simulink model "VCU_SW"  (R2020b)
settings: Solver=FixedStepDiscrete  StartTime=0.0  StopTime=inf  FixedStep=1e-2  RelTol=1e-3
PreLoadFcn:
  | RTWConfigurationCB('preloadfcn', bdroot);
InitFcn:
  | loadvar_ttc500
undefined symbols (not defined in the file or in its folder): BrkPedalTypes, CabMovModeTypes, cFuseTempSensAcc_X, cFuseTempSensAcc_Y, cFuseTempSensVal_X, cFuseTempSensVal_Y, cTMSTempSensVal_X, cTMSTempSensVal_Y, cTransferCaseSpeedRatio, diag_state, DoorsPositionTypes, dP_filter_Y, DriverOccClassSystemTypes, ErrorValueTypes, fatal_error_callback, IO_ADC_NO_RANGE, LadderStatusTypes, pAnalogCabRotSensAcc, pAnalogCabRotSensMaxVolt, pAnalogCabRotSensMinVolt, pAnalogCabRotSensRange, pAnalogCabRotSensZeroVolt, pBrkActivePress, pCabTiltSensAcc, pCabTiltSensMaxCur, pCabTiltSensMinCur, pDistanceCorrection, pECANManual_BPNEnable, pECANManual_BPNEnabler_Flag, pFilterSensAccRes, pHDirMaxDiffFrq, pHDirSensHighLvl, pHDirSensLowLvl, pMainGearRatio, pMaxFilterSensRes, pMaxFirstPedalSensValue, pMaxFuseTempSensRes, pMaxPressLoss, pMaxPressSensCurrent, pMaxPressValue, pMaxPressValueHydMotAndPump, pMaxPressValueParkDrain, pMaxSecondPedalSensValue, pMaxTempSensVoltage, pMaxTempValue, pMaxTMSTempSensRes, pMinFilterSensRes, pMinFirstPedalSensValue, pMinFuseTempSensRes, pMinPressLoss, pMinPressSensCurrent, pMinPressValue, pMinSecondPedalSensValue, pMinTempSensVoltage, pMinTempValue, pMinTMSTempSensRes, pMotorRingTeethNum, pPedalSensAccuracyPct, pPedalSensAccuracyVolt, pPressLossTreshhold ... (+20)
libraries: TTlibrary x271, canmsglib x128, simulink x88
(part 8 of 17)

== system VCU_SW/OutputLayer/OutputNetwork/OutputCCAN/SetCCAN100msec ==
  function : TriggerPort  TriggerType=function-call  VariantControl=Variant
  CANPack_DCDC_IN_Control : canmsglib/CAN Pack  Commented=on  CANdbFile=C:\Users\shevchenko\Desktop\HerculesLittle\HerculesLittle\database\ElectricCAN.dbc  MsgList=(none)  MsgName=DCDC_IN_Control  MsgIDType=Extended (29-bit identifier)  MsgIdentifier=73  MsgLength=8  Remote=off  ApplyMinMax=off  BusOutput=on  SignalInfo={'BPN_Enable','0','1','LE','unsigned','Standard','0','1','0','0','1'}
      settings: SourceProductBaseCode=ME,XP,VN  DataFormat=CANdb specified signals
  CANPack_DCDC_IN_Control1 : canmsglib/CAN Pack  Commented=on  MsgList=(none)  MsgName=ETC2  MsgIDType=Extended (29-bit identifier)  MsgIdentifier=418383354  MsgLength=8  Remote=off  ApplyMinMax=off  BusOutput=on  SignalInfo={ 'Transmission_Actual_Gear_Ratio', '8', '16', 'LE', 'unsigned', 'Standard', '0', '0.001', '0', '0', '64.255'; 'Transmission_Current_Gear', '24', '8', 'LE', 'unsigned', 'Standard', '0', '1', '-125', '-125', '125'; 'Transmission_Current_Range', '48', '16', 'LE', 'unsigned', 'Standard', '0', '1', '0', '0', '65535'; 'Transmission_Requested_Range', '32', '16', 'LE', 'unsigned', 'Standard', '0', '1', '0', '0', '65535'; 'Transmission_Selected_Gear', '0', '8', 'LE', 'unsigned', 'Standard', '0', '1', '-125', '-125', '125' }
      settings: SourceProductBaseCode=ME,XP,VN  DataFormat=manually specified signals
  CCVS1 : Subsystem
  Cabine Angles : Subsystem
  "Cabine Status " : Subsystem
  Constant31 : Constant  Commented=on  Value=pECANManual_BPNEnabler_Flag
  Constant32 : Constant  Commented=on  Value=pECANManual_BPNEnable
  Data Store Read : DataStoreRead  Commented=on  DataStoreName=OutputNetworkData  DataStoreElements=DevicesControllerData.ovc_permission
  Data Store Read1 : DataStoreRead  Commented=on  DataStoreName=OutputNetworkData  DataStoreElements=DevicesControllerData.ovc_permission
  EBC1 : Subsystem
  ETC2 : Subsystem
  ETC7 : Subsystem
  "Fuel Filter Heater Status " : Subsystem
  FuelUsingOEM : Subsystem
  MATLAB Function6 : MATLAB Function  Commented=on  TreatAsAtomicUnit=on
  Multiport Switch5 : MultiPortSwitch  Commented=on  DataPortOrder=Zero-based contiguous  Inputs=2  zeroidx=on
  Terminator : Terminator  Commented=on
  Terminator1 : Terminator  Commented=on
  VD : Subsystem
  "VLVCMD_ MANIP_TABLE " : Subsystem
  transmit_message_dcdc_in_control : TTlibrary/CAN/transmit_message_name  Commented=on  channel=IO_CAN_CHANNEL_0  id_format=IO_CAN_STD_FRAME  retranslation=off  io_error=on  sample_time=-1
      settings: SourceProductName=TT control 500 series
  transmit_message_dcdc_in_control1 : TTlibrary/CAN/transmit_message_name  Commented=on  channel=IO_CAN_CHANNEL_1  id_format=IO_CAN_STD_FRAME  retranslation=off  io_error=on  sample_time=-1
      settings: SourceProductName=TT control 500 series
  wires:
  Data Store Read1/1 -> CANPack_DCDC_IN_Control1/1
  transmit_message_dcdc_in_control1/1 -> Terminator1/1  "error_tx_transmit_message_dcdc_in_control1"
  CANPack_DCDC_IN_Control1/1 -> transmit_message_dcdc_in_control1/1
  Data Store Read/1 -> MATLAB Function6/1(input)
  transmit_message_dcdc_in_control/1 -> Terminator/1  "error_tx_transmit_message_dcdc_in_control"
  MATLAB Function6/1(value) -> Multiport Switch5/2
  Multiport Switch5/1 -> CANPack_DCDC_IN_Control/1
  Constant32/1 -> Multiport Switch5/3
  CANPack_DCDC_IN_Control/1 -> transmit_message_dcdc_in_control/1
  Constant31/1 -> Multiport Switch5/1

== system VCU_SW/OutputLayer/OutputNetwork/OutputCCAN/SetCCAN10msec ==
  function : TriggerPort  TriggerType=function-call  VariantControl=Variant

== system VCU_SW/OutputLayer/OutputNetwork/OutputCCAN/SetCCAN500msec ==
  function : TriggerPort  TriggerType=function-call  VariantControl=Variant
  Brake_circuits_manip_press : Subsystem
  CANPack_DCDC_IN_Control : canmsglib/CAN Pack  Commented=on  CANdbFile=C:\Users\shevchenko\Desktop\HerculesLittle\HerculesLittle\database\ElectricCAN.dbc  MsgList=(none)  MsgName=DCDC_IN_Control  MsgIDType=Extended (29-bit identifier)  MsgIdentifier=73  MsgLength=8  Remote=off  ApplyMinMax=off  BusOutput=on  SignalInfo={'BPN_Enable','0','1','LE','unsigned','Standard','0','1','0','0','1'}
      settings: SourceProductBaseCode=ME,XP,VN  DataFormat=CANdb specified signals
  CANPack_DCDC_IN_Control1 : canmsglib/CAN Pack  Commented=on  MsgList=(none)  MsgName=ETC2  MsgIDType=Extended (29-bit identifier)  MsgIdentifier=418383354  MsgLength=8  Remote=off  ApplyMinMax=off  BusOutput=on  SignalInfo={ 'Transmission_Actual_Gear_Ratio', '8', '16', 'LE', 'unsigned', 'Standard', '0', '0.001', '0', '0', '64.255'; 'Transmission_Current_Gear', '24', '8', 'LE', 'unsigned', 'Standard', '0', '1', '-125', '-125', '125'; 'Transmission_Current_Range', '48', '16', 'LE', 'unsigned', 'Standard', '0', '1', '0', '0', '65535'; 'Transmission_Requested_Range', '32', '16', 'LE', 'unsigned', 'Standard', '0', '1', '0', '0', '65535'; 'Transmission_Selected_Gear', '0', '8', 'LE', 'unsigned', 'Standard', '0', '1', '-125', '-125', '125' }
      settings: SourceProductBaseCode=ME,XP,VN  DataFormat=manually specified signals
  Constant31 : Constant  Commented=on  Value=pECANManual_BPNEnabler_Flag
  Constant32 : Constant  Commented=on  Value=pECANManual_BPNEnable
  Data Store Read : DataStoreRead  Commented=on  DataStoreName=OutputNetworkData  DataStoreElements=DevicesControllerData.ovc_permission
  Data Store Read1 : DataStoreRead  Commented=on  DataStoreName=OutputNetworkData  DataStoreElements=DevicesControllerData.ovc_permission
  EAC1 : Subsystem
  "EFL/P1 " : Subsystem
  EFL/P12 : Subsystem  Commented=on
  MATLAB Function6 : MATLAB Function  Commented=on  TreatAsAtomicUnit=on
  Multiport Switch5 : MultiPortSwitch  Commented=on  DataPortOrder=Zero-based contiguous  Inputs=2  zeroidx=on
  Terminator : Terminator  Commented=on
  Terminator1 : Terminator  Commented=on
  transmit_message_dcdc_in_control : TTlibrary/CAN/transmit_message_name  Commented=on  channel=IO_CAN_CHANNEL_0  id_format=IO_CAN_STD_FRAME  retranslation=off  io_error=on  sample_time=-1
      settings: SourceProductName=TT control 500 series
  transmit_message_dcdc_in_control1 : TTlibrary/CAN/transmit_message_name  Commented=on  channel=IO_CAN_CHANNEL_1  id_format=IO_CAN_STD_FRAME  retranslation=off  io_error=on  sample_time=-1
      settings: SourceProductName=TT control 500 series
  wires:
  transmit_message_dcdc_in_control1/1 -> Terminator1/1  "error_tx_transmit_message_dcdc_in_control1"
  Data Store Read1/1 -> CANPack_DCDC_IN_Control1/1
  CANPack_DCDC_IN_Control1/1 -> transmit_message_dcdc_in_control1/1
  Data Store Read/1 -> MATLAB Function6/1(input)
  transmit_message_dcdc_in_control/1 -> Terminator/1  "error_tx_transmit_message_dcdc_in_control"
  MATLAB Function6/1(value) -> Multiport Switch5/2
  Multiport Switch5/1 -> CANPack_DCDC_IN_Control/1
  Constant32/1 -> Multiport Switch5/3
  CANPack_DCDC_IN_Control/1 -> transmit_message_dcdc_in_control/1
  Constant31/1 -> Multiport Switch5/1

== system VCU_SW/OutputLayer/OutputNetwork/OutputCCAN/SetCCAN50msec ==
  function : TriggerPort  TriggerType=function-call  VariantControl=Variant
  EEC1 : Subsystem
  EEC2 : Subsystem

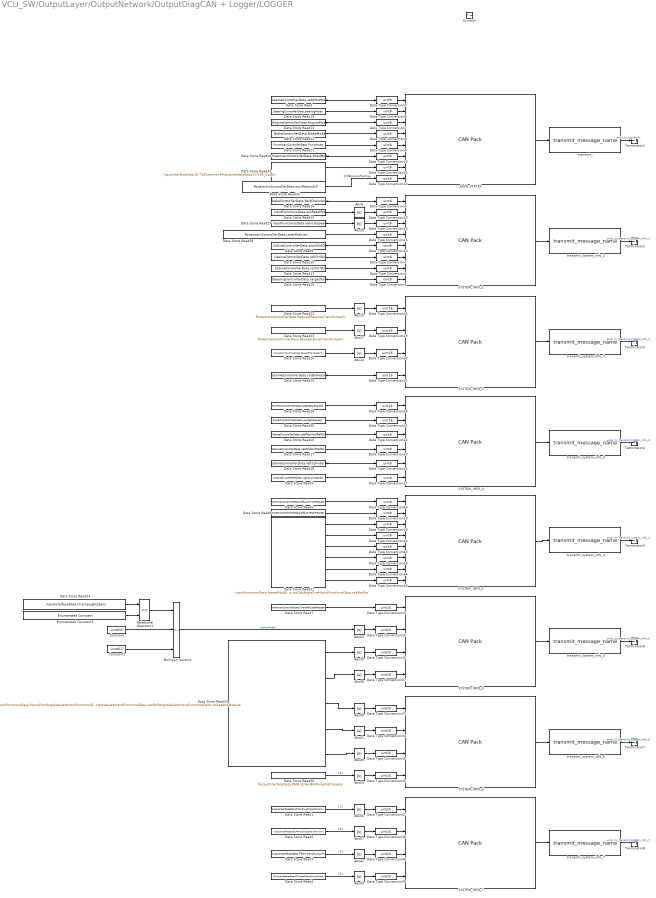
== system VCU_SW/OutputLayer/OutputNetwork/OutputDiagCAN + Logger/LOGGER ==
  function : TriggerPort  TriggerType=function-call  VariantControl=Variant
  ALGO_STATES : canmsglib/CAN Pack  MsgList=(none)  MsgName=ALGO_STATES  MsgIDType=Extended (29-bit identifier)  MsgIdentifier=419385594  MsgLength=8  Remote=off  ApplyMinMax=off  BusOutput=on  SignalInfo={ 'ALGO_MODE_1', '56', '8', 'LE', 'unsigned', 'Standard', '0', '1', '0', '0', '255'; 'ALGO_MODE_2', '48', '8', 'LE', 'unsigned', 'Standard', '0', '1', '0', '0', '255'; 'ALGO_MODE_3', '40', '8', 'LE', 'unsigned', 'Standard', '0', '1', '0', '0', '255'; 'ALGO_MODE_4', '32', '8', 'LE', 'unsigned', 'Standard', '0', '1', '0', '0', '255'; 'ALGO_MODE_5', '24', '8', 'LE', 'unsigned', 'Standard', '0', '1', '0', '0', '255'; 'ALGO_MODE_6', '16', '8', 'LE', 'unsigned', 'Standard', '0', '1', '0', '0', '255'; 'ALGO_MODE_7', '8', '8', 'LE', 'unsigned', 'Standard', '0', '1', '0', '0', '255'; 'ALGO_MODE_8', '0', '8', 'LE', 'unsigned', 'Standard', '0', '1', '0', '0', '255' }
      settings: SourceProductBaseCode=ME,XP,VN  DataFormat=manually specified signals
  Abs{9..10,16..17,24,34..35,40..43,49..50,56..57,63} (16 alike) : Abs
  Constant : Constant  Value=uint8(0)
  Constant1 : Constant  Value=uint8(1)
  Data Store Read : DataStoreRead  DataStoreName=CabineControllerData  DataStoreElements=CabineControllerData.cabMovMode
  Data Store Read1 : DataStoreRead  DataStoreName=OutputInterfaceData  DataStoreElements=OutputInterfaceData.PWM.driveTransPumpVlv
  Data Store Read10 : DataStoreRead  DataStoreName=CabineControllerData  DataStoreElements=CabineControllerData.rollCtrlDir
  Data Store Read11 : DataStoreRead  DataStoreName=CabineControllerData  DataStoreElements=CabineControllerData.rotCtrlDir
  Data Store Read12 : DataStoreRead  DataStoreName=EngineControllerData  DataStoreElements=EngineControllerData.EngineMode
  Data Store Read13 : DataStoreRead  DataStoreName=BrakeControllerData  DataStoreElements=BrakeControllerData.BrakeMode
  Data Store Read14 : DataStoreRead  DataStoreName=BrakeControllerData  DataStoreElements=BrakeControllerData.ParkDrainValve
  Data Store Read15 : DataStoreRead  DataStoreName=InputFunctionsData  DataStoreElements=InputFunctionsData.accPedalPos
  Data Store Read16 : DataStoreRead  DataStoreName=CabineControllerData  DataStoreElements=CabineControllerData.cabPitchHullRefDir
  Data Store Read17 : DataStoreRead  DataStoreName=CabineControllerData  DataStoreElements=CabineControllerData.cabRollHullRefDir
  Data Store Read18 : DataStoreRead  DataStoreName=CabineControllerData  DataStoreElements=CabineControllerData.leftCylinderDir
  Data Store Read19 : DataStoreRead  DataStoreName=SteeringControllerData  DataStoreElements=SteeringControllerData.steeringMode
  Data Store Read2 : DataStoreRead  DataStoreName=OutputInterfaceData  DataStoreElements=OutputInterfaceData.PWM.reverseTransPumpVlv
  Data Store Read20 : DataStoreRead  DataStoreName=PowertrainControllerData  DataStoreElements=PowertrainControllerData.RoadMode
  Data Store Read21 : DataStoreRead  DataStoreName=PowertrainControllerData  DataStoreElements=PowertrainControllerData.PumpMode
  Data Store Read22 : DataStoreRead  DataStoreName=PowertrainControllerData  DataStoreElements=PowertrainControllerData.RequestReverseTransPumpVlv
  Data Store Read23 : DataStoreRead  DataStoreName=PowertrainControllerData  DataStoreElements=PowertrainControllerData.RequestDriveTransPumpVlv
  Data Store Read24 : DataStoreRead  DataStoreName=PowertrainControllerData  DataStoreElements=PowertrainControllerData.RequestTransMotorVlv
  Data Store Read25 : DataStoreRead  DataStoreName=CabineControllerData  DataStoreElements=CabineControllerData.rotBrakeCmd
  Data Store Read26 : DataStoreRead  DataStoreName=SteeringControllerData  DataStoreElements=SteeringControllerData.targetValve
  Data Store Read27 : DataStoreRead  DataStoreName=InputFunctionsData  DataStoreElements=InputFunctionsData.vehicleSpeed
  Data Store Read28 : DataStoreRead  DataStoreName=PowertrainControllerData  DataStoreElements=PowertrainControllerData.LeverPosition
  Data Store Read29 : DataStoreRead  DataStoreName=PowertrainControllerData  DataStoreElements=PowertrainControllerData.UpperGearRequest
  Data Store Read3 : DataStoreRead  DataStoreName=OutputInterfaceData  DataStoreElements=OutputInterfaceData.PWM.transPumpVlv
  Data Store Read30 : DataStoreRead  DataStoreName=PowertrainControllerData  DataStoreElements=PowertrainControllerData.LowGearRequest
  Data Store Read31 : DataStoreRead  DataStoreName=InputFunctionsData  DataStoreElements=InputFunctionsData.framePitchAngleDir#InputFunctionsData.frameRollAngleDir#InputFunctionsData.cabPitchAngleDir#InputFunctionsData.cabRollAngleDir#InputFunctionsData.rotCabAngleDir#InputFunctionsData.cabRotPos
  Data Store Read32 : DataStoreRead  DataStoreName=InputFunctionsData  DataStoreElements=InputFunctionsData.framePitchAngleValue#InputFunctionsData.frameRollAngleValue#InputFunctionsData.cabPitchAngleValue#InputFunctionsData.cabRollAngleValue#InputFunctionsData.rotCabAngleValue
  Data Store Read33 : DataStoreRead  DataStoreName=InputInterfaceData  DataStoreElements=InputInterfaceData.DI.T15Common#InputInterfaceData.DI.T50_Supply
  Data Store Read34 : DataStoreRead  DataStoreName=InputInterfaceData  DataStoreElements=InputInterfaceData.DI.stopLightsSens
  Data Store Read35 : DataStoreRead  DataStoreName=PowertrainControllerData  DataStoreElements=PowertrainControllerData.movRestrictLP
  Data Store Read36 : DataStoreRead  DataStoreName=OutputInterfaceData  DataStoreElements=OutputInterfaceData.PWM.strAndBrkPumpDistrSupply
  Data Store Read4 : DataStoreRead  DataStoreName=OutputInterfaceData  DataStoreElements=OutputInterfaceData.PWM.techEquipPumpSupply
  Data Store Read5 : DataStoreRead  DataStoreName=PowertrainControllerData  DataStoreElements=PowertrainControllerData.DiffLockFrontRequest
  Data Store Read6 : DataStoreRead  DataStoreName=PowertrainControllerData  DataStoreElements=PowertrainControllerData.DiffLockRearRequest
  Data Store Read7 : DataStoreRead  DataStoreName=PowertrainControllerData  DataStoreElements=PowertrainControllerData.TransferCaseRequest
  Data Store Read8 : DataStoreRead  DataStoreName=CabineControllerData  DataStoreElements=CabineControllerData.pitchCtrlDir
  Data Store Read9 : DataStoreRead  DataStoreName=CabineControllerData  DataStoreElements=CabineControllerData.rightCylinderDir
  Data Type Conversion{1..20,22..24,42..46} (28 alike) : DataTypeConversion  OutDataTypeStr=uint8
  Data Type Conversion{21,25..41} (18 alike) : DataTypeConversion  OutDataTypeStr=uint16
  Enumerated Constant5 : simulink/Sources/Enumerated Constant  OutDataTypeStr=Enum: StateModeTypes  Value=StateModeTypes.STT_ENABLE  SampleTime=inf
  Multiport Switch2 : MultiPortSwitch  DataPortOrder=Zero-based contiguous  Inputs=2  zeroidx=on
  Relational Operator1 : RelationalOperator  Operator===  OutDataTypeStr=boolean  RndMeth=Simplest
  SYSTEM_INFO_1 : canmsglib/CAN Pack  MsgList=(none)  MsgName=SYSTEM_INFO_1  MsgIDType=Extended (29-bit identifier)  MsgIdentifier=419387642  MsgLength=8  Remote=off  ApplyMinMax=off  BusOutput=on  SignalInfo={ 'system_info_1_1', '0', '8', 'LE', 'unsigned', 'Standard', '0', '1', '0', '0', '255'; 'system_info_1_2', '8', '8', 'LE', 'unsigned', 'Standard', '0', '1', '0', '0', '255'; 'system_info_1_3', '16', '8', 'LE', 'unsigned', 'Standard', '0', '1', '0', '0', '255'; 'system_info_1_4', '24', '8', 'LE', 'unsigned', 'Standard', '0', '1', '0', '0', '255'; 'system_info_1_5', '32', '8', 'LE', 'unsigned', 'Standard', '0', '1', '0', '0', '255'; 'system_info_1_6', '40', '8', 'LE', 'unsigned', 'Standard', '0', '1', '0', '0', '255'; 'system_info_1_7', '48', '8', 'LE', 'unsigned', 'Standard', '0', '1', '0', '0', '255'; 'system_info_1_8', '56', '8', 'LE', 'unsigned', 'Standard', '0', '1', '0', '0', '255' }
      settings: SourceProductBaseCode=ME,XP,VN  DataFormat=manually specified signals
  SYSTEM_INFO_2 : canmsglib/CAN Pack  MsgList=(none)  MsgName=SYSTEM_INFO_2  MsgIDType=Extended (29-bit identifier)  MsgIdentifier=419387898  MsgLength=8  Remote=off  ApplyMinMax=off  BusOutput=on  SignalInfo={ 'system_info_2_1', '0', '16', 'LE', 'unsigned', 'Standard', '0', '1', '0', '0', '65535'; 'system_info_2_2', '16', '16', 'LE', 'unsigned', 'Standard', '0', '1', '0', '0', '65535'; 'system_info_2_3', '32', '16', 'LE', 'unsigned', 'Standard', '0', '1', '0', '0', '65535'; 'system_info_2_4', '48', '16', 'LE', 'unsigned', 'Standard', '0', '1', '0', '0', '65535' }
      settings: SourceProductBaseCode=ME,XP,VN  DataFormat=manually specified signals
  SYSTEM_INFO_3 : canmsglib/CAN Pack  MsgList=(none)  MsgName=SYSTEM_INFO_3  MsgIDType=Extended (29-bit identifier)  MsgIdentifier=419389690  MsgLength=8  Remote=off  ApplyMinMax=off  BusOutput=on  SignalInfo={ 'system_info_3_1', '0', '16', 'LE', 'unsigned', 'Standard', '0', '1', '0', '0', '65535'; 'system_info_3_3', '16', '16', 'LE', 'unsigned', 'Standard', '0', '1', '0', '0', '65535'; 'system_info_3_5', '32', '8', 'LE', 'unsigned', 'Standard', '0', '1', '0', '0', '255'; 'system_info_3_6', '40', '8', 'LE', 'unsigned', 'Standard', '0', '1', '0', '0', '255'; 'system_info_3_7', '48', '8', 'LE', 'unsigned', 'Standard', '0', '1', '0', '0', '255'; 'system_info_3_8', '56', '8', 'LE', 'unsigned', 'Standard', '0', '1', '0', '0', '255' }
      settings: SourceProductBaseCode=ME,XP,VN  DataFormat=manually specified signals
  SYSTEM_INFO_4 : canmsglib/CAN Pack  MsgList=(none)  MsgName=SYSTEM_INFO_4  MsgIDType=Extended (29-bit identifier)  MsgIdentifier=419389946  MsgLength=8  Remote=off  ApplyMinMax=off  BusOutput=on  SignalInfo={ 'system_info_4_1', '0', '8', 'LE', 'unsigned', 'Standard', '0', '1', '0', '0', '255'; 'system_info_4_2', '8', '8', 'LE', 'unsigned', 'Standard', '0', '1', '0', '0', '255'; 'system_info_4_3', '16', '8', 'LE', 'unsigned', 'Standard', '0', '1', '0', '0', '255'; 'system_info_4_4', '24', '8', 'LE', 'unsigned', 'Standard', '0', '1', '0', '0', '255'; 'system_info_4_5', '32', '8', 'LE', 'unsigned', 'Standard', '0', '1', '0', '-Inf', 'Inf'; 'system_info_4_6', '40', '8', 'LE', 'unsigned', 'Standard', '0', '1', '0', '-Inf', 'Inf'; 'system_info_4_7', '48', '8', 'LE', 'unsigned', 'Standard', '0', '1', '0', '-Inf', 'Inf'; 'system_info_4_8', '56', '8', 'LE', 'unsigned', 'Standard', '0', '1', '0', '-Inf', 'Inf' }
      settings: SourceProductBaseCode=ME,XP,VN  DataFormat=manually specified signals
  SYSTEM_INFO_5 : canmsglib/CAN Pack  MsgList=(none)  MsgName=SYSTEM_INFO_5  MsgIDType=Extended (29-bit identifier)  MsgIdentifier=419390202  MsgLength=8  Remote=off  ApplyMinMax=off  BusOutput=on  SignalInfo={ 'system_info_5_1', '0', '16', 'LE', 'unsigned', 'Standard', '0', '1', '0', '0', '65535'; 'system_info_5_2', '16', '16', 'LE', 'unsigned', 'Standard', '0', '1', '0', '0', '65535'; 'system_info_5_3', '32', '16', 'LE', 'unsigned', 'Standard', '0', '1', '0', '0', '65535'; 'system_info_5_4', '48', '16', 'LE', 'unsigned', 'Standard', '0', '1', '0', '0', '65535' }
      settings: SourceProductBaseCode=ME,XP,VN  DataFormat=manually specified signals
  SYSTEM_INFO_6 : canmsglib/CAN Pack  MsgList=(none)  MsgName=SYSTEM_INFO_6  MsgIDType=Extended (29-bit identifier)  MsgIdentifier=419390458  MsgLength=8  Remote=off  ApplyMinMax=off  BusOutput=on  SignalInfo={ 'system_info_6_1', '0', '16', 'LE', 'unsigned', 'Standard', '0', '1', '0', '0', '65535'; 'system_info_6_2', '16', '16', 'LE', 'unsigned', 'Standard', '0', '1', '0', '0', '65535'; 'system_info_6_3', '32', '16', 'LE', 'unsigned', 'Standard', '0', '1', '0', '0', '65535'; 'system_info_6_4', '48', '16', 'LE', 'unsigned', 'Standard', '0', '1', '0', '0', '65535' }
      settings: SourceProductBaseCode=ME,XP,VN  DataFormat=manually specified signals
  SYSTEM_INFO_7 : canmsglib/CAN Pack  MsgList=(none)  MsgName=SYSTEM_INFO_7  MsgIDType=Extended (29-bit identifier)  MsgIdentifier=419391226  MsgLength=8  Remote=off  ApplyMinMax=off  BusOutput=on  SignalInfo={ 'system_info_7_1', '0', '16', 'LE', 'unsigned', 'Standard', '0', '1', '0', '0', '65535'; 'system_info_7_2', '16', '16', 'LE', 'unsigned', 'Standard', '0', '1', '0', '0', '65535'; 'system_info_7_3', '32', '16', 'LE', 'unsigned', 'Standard', '0', '1', '0', '0', '65535'; 'system_info_7_4', '48', '16', 'LE', 'unsigned', 'Standard', '0', '1', '0', '0', '65535' }
      settings: SourceProductBaseCode=ME,XP,VN  DataFormat=manually specified signals
  Terminator{1..8} (8 alike) : Terminator
  transmit_ : TTlibrary/CAN/transmit_message_name  channel=IO_CAN_CHANNEL_6  id_format=IO_CAN_EXT_FRAME  retranslation=off  io_error=on  sample_time=-1
      settings: SourceProductName=TT control 500 series
  transmit_system_info_{1..7} (7 alike) : TTlibrary/CAN/transmit_message_name  channel=IO_CAN_CHANNEL_6  id_format=IO_CAN_EXT_FRAME  retranslation=off  io_error=on  sample_time=-1
      settings: SourceProductName=TT control 500 series
  wires:
  Data Type Conversion6/1 -> ALGO_STATES/2
  Data Store Read13/1 -> Data Type Conversion8/1
  Data Store Read12/1 -> Data Type Conversion7/1
  Data Store Read33/1 -> Data Type Conversion11/1
  Data Store Read19/1 -> Data Type Conversion6/1
  Data Store Read/1 -> Data Type Conversion3/1
  Data Store Read20/1 -> Data Type Conversion10/1
  Data Store Read21/1 -> Data Type Conversion9/1
  ALGO_STATES/1 -> transmit_/1
  Data Type Conversion12/1 -> ALGO_STATES/8
  Data Type Conversion11/1 -> ALGO_STATES/7
  Data Type Conversion3/1 -> ALGO_STATES/1
  Data Type Conversion9/1 -> ALGO_STATES/5
  Data Type Conversion7/1 -> ALGO_STATES/3
  Data Type Conversion8/1 -> ALGO_STATES/4
  transmit_/1 -> Terminator1/1  "error_tx_transmit_"
  Data Type Conversion10/1 -> ALGO_STATES/6
  Data Type Conversion1/1 -> SYSTEM_INFO_1/6
  transmit_system_info_1/1 -> Terminator2/1  "error_tx_transmit_system_info_1"
  Data Type Conversion15/1 -> SYSTEM_INFO_1/4
  Data Type Conversion14/1 -> SYSTEM_INFO_1/3
  Data Type Conversion16/1 -> SYSTEM_INFO_1/5
  Data Type Conversion5/1 -> SYSTEM_INFO_1/1
  Data Type Conversion2/1 -> SYSTEM_INFO_1/7
  Data Type Conversion4/1 -> SYSTEM_INFO_1/8
  SYSTEM_INFO_1/1 -> transmit_system_info_1/1
  Data Store Read8/1 -> Data Type Conversion16/1
  Data Store Read10/1 -> Data Type Conversion1/1
  Data Store Read14/1 -> Data Type Conversion5/1
  Abs9/1 -> Data Type Conversion13/1
  Data Store Read26/1 -> Data Type Conversion4/1
  Data Store Read11/1 -> Data Type Conversion2/1
  Abs10/1 -> Data Type Conversion14/1
  Data Store Read28/1 -> Data Type Conversion15/1
  Data Type Conversion13/1 -> SYSTEM_INFO_1/2
  Data Type Conversion21/1 -> SYSTEM_INFO_3/2
  Data Store Read17/1 -> Data Type Conversion23/1
  Data Store Read16/1 -> Data Type Conversion22/1
  Data Store Read30/1 -> Data Type Conversion21/1
  Data Store Read29/1 -> Data Type Conversion28/1
  Data Store Read9/1 -> Data Type Conversion17/1
  Data Store Read18/1 -> Data Type Conversion24/1
  SYSTEM_INFO_3/1 -> transmit_system_info_3/1
  Data Type Conversion28/1 -> SYSTEM_INFO_3/1
  Data Type Conversion24/1 -> SYSTEM_INFO_3/5
  Data Type Conversion22/1 -> SYSTEM_INFO_3/3
  Data Type Conversion23/1 -> SYSTEM_INFO_3/4
  transmit_system_info_3/1 -> Terminator4/1  "error_tx_transmit_system_info_3"
  Data Type Conversion17/1 -> SYSTEM_INFO_3/6
  transmit_system_info_2/1 -> Terminator3/1  "error_tx_transmit_system_info_2"
  Data Type Conversion31/1 -> SYSTEM_INFO_2/4
  Data Type Conversion30/1 -> SYSTEM_INFO_2/3
  Data Type Conversion26/1 -> SYSTEM_INFO_2/1
  SYSTEM_INFO_2/1 -> transmit_system_info_2/1
  Abs16/1 -> Data Type Conversion26/1
  Abs17/1 -> Data Type Conversion29/1
  Abs24/1 -> Data Type Conversion30/1
  Data Store Read25/1 -> Data Type Conversion31/1
  Data Type Conversion29/1 -> SYSTEM_INFO_2/2
  Data Type Conversion34/1 -> SYSTEM_INFO_6/2
  Abs50/1 -> Data Type Conversion35/1
  Abs49/1 -> Data Type Conversion36/1
  Abs41/1 -> Data Type Conversion34/1
  Abs40/1 -> Data Type Conversion37/1
  SYSTEM_INFO_6/1 -> transmit_system_info_6/1
  Data Type Conversion37/1 -> SYSTEM_INFO_6/1
  Data Type Conversion36/1 -> SYSTEM_INFO_6/3
  Data Type Conversion35/1 -> SYSTEM_INFO_6/4
  transmit_system_info_6/1 -> Terminator7/1  "error_tx_transmit_system_info_6"
  transmit_system_info_7/1 -> Terminator8/1  "error_tx_transmit_system_info_7"
  Data Type Conversion39/1 -> SYSTEM_INFO_7/4
  Data Type Conversion40/1 -> SYSTEM_INFO_7/3
  Data Type Conversion41/1 -> SYSTEM_INFO_7/1
  SYSTEM_INFO_7/1 -> transmit_system_info_7/1
  Abs56/1 -> Data Type Conversion41/1
  Abs57/1 -> Data Type Conversion38/1
  Abs42/1 -> Data Type Conversion40/1
  Abs43/1 -> Data Type Conversion39/1
  Data Type Conversion38/1 -> SYSTEM_INFO_7/2
  Data Type Conversion25/1 -> SYSTEM_INFO_5/2
  Abs35/1 -> Data Type Conversion27/1
  Abs34/1 -> Data Type Conversion32/1
  Abs63/1 -> Data Type Conversion25/1
  Data Store Read7/1 -> Data Type Conversion33/1
  SYSTEM_INFO_5/1 -> transmit_system_info_5/1
  Data Type Conversion33/1 -> SYSTEM_INFO_5/1
  Data Type Conversion32/1 -> SYSTEM_INFO_5/3
  Data Type Conversion27/1 -> SYSTEM_INFO_5/4
  transmit_system_info_5/1 -> Terminator6/1  "error_tx_transmit_system_info_5"
  transmit_system_info_4/1 -> Terminator5/1  "error_tx_transmit_system_info_4"
  SYSTEM_INFO_4/1 -> transmit_system_info_4/1
  Data Store Read15/1 -> Abs9/1
  Data Store Read27/1 -> Abs10/1
  Data Store Read1/1 -> Abs56/1  "101"
  Data Store Read2/1 -> Abs57/1  "102"
  Data Store Read3/1 -> Abs42/1  "126"
  Data Store Read4/1 -> Abs43/1  "154"
  Data Store Read36/1 -> Abs50/1  "184"
  Data Store Read22/1 -> Abs16/1
  Data Store Read23/1 -> Abs17/1
  Data Store Read24/1 -> Abs24/1
  Data Store Read31/6 -> Data Type Conversion45/1
  Data Store Read6/1 -> Data Type Conversion19/1
  Data Store Read31/4 -> Data Type Conversion18/1
  Data Store Read5/1 -> Data Type Conversion46/1
  Data Store Read31/1 -> Data Type Conversion20/1
  Data Store Read31/5 -> Data Type Conversion44/1
  Data Store Read31/2 -> Data Type Conversion42/1
  Data Type Conversion46/1 -> SYSTEM_INFO_4/1
  Data Type Conversion42/1 -> SYSTEM_INFO_4/4
  Data Store Read31/3 -> Data Type Conversion43/1
  Data Type Conversion44/1 -> SYSTEM_INFO_4/7
  Data Type Conversion43/1 -> SYSTEM_INFO_4/5
  Data Type Conversion20/1 -> SYSTEM_INFO_4/3
  Data Type Conversion45/1 -> SYSTEM_INFO_4/8
  Data Type Conversion18/1 -> SYSTEM_INFO_4/6
  Data Type Conversion19/1 -> SYSTEM_INFO_4/2
  Data Store Read32/1 -> Abs34/1
  Data Store Read32/5 -> Abs49/1
  Data Store Read32/4 -> Abs41/1
  Data Store Read32/3 -> Abs40/1
  Data Store Read32/2 -> Abs35/1
  Constant/1 -> Multiport Switch2/2
  Constant1/1 -> Multiport Switch2/3
  Enumerated Constant5/1 -> Relational Operator1/2
  Relational Operator1/1 -> Multiport Switch2/1
  Multiport Switch2/1 -> Abs63/1  "brakePedal"
  Data Store Read34/1 -> Relational Operator1/1
  Data Store Read35/1 -> Data Type Conversion12/1  "DiffBlockAccPedFlag"

== system VCU_SW/OutputLayer/OutputNetwork/OutputDiagCAN + Logger/SetDiagCAN10msec ==
  function : TriggerPort  TriggerType=function-call  VariantControl=Variant
  Data Store Read : DataStoreRead  DataStoreName=UDSStruct  DataStoreElements=UDSStruct.readUDSmsgFlag
  MATLAB Function : MATLAB Function  TreatAsAtomicUnit=on
  Simulink Function : Subsystem  TreatAsAtomicUnit=on
  wires:
  Data Store Read/1 -> MATLAB Function/1(flag)

== system VCU_SW/OutputLayer/OutputNetwork/OutputDiagCAN + Logger/SetDiagCAN10msec1 ==
  function : TriggerPort  TriggerType=function-call  VariantControl=Variant
  Data Store Read : DataStoreRead  DataStoreName=UDSStruct  DataStoreElements=UDSStruct.readUDSmsgFlag
  MATLAB Function : MATLAB Function  TreatAsAtomicUnit=on
  Simulink Function : Subsystem  TreatAsAtomicUnit=on
  wires:
  Data Store Read/1 -> MATLAB Function/1(readflag)

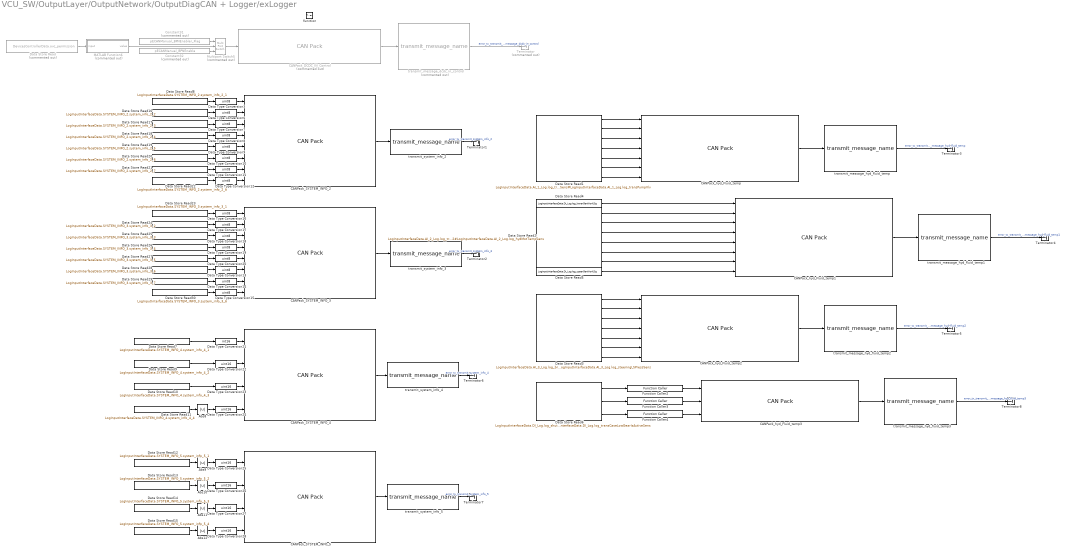
== system VCU_SW/OutputLayer/OutputNetwork/OutputDiagCAN + Logger/exLogger ==
  function : TriggerPort  TriggerType=function-call  VariantControl=Variant
  Abs{8..12} (5 alike) : Abs
  CANPack_DCDC_IN_Control : canmsglib/CAN Pack  Commented=on  CANdbFile=C:\Users\shevchenko\Desktop\HerculesLittle\HerculesLittle\database\ElectricCAN.dbc  MsgList=(none)  MsgName=DCDC_IN_Control  MsgIDType=Extended (29-bit identifier)  MsgIdentifier=73  MsgLength=8  Remote=off  ApplyMinMax=off  BusOutput=on  SignalInfo={'BPN_Enable','0','1','LE','unsigned','Standard','0','1','0','0','1'}
      settings: SourceProductBaseCode=ME,XP,VN  DataFormat=CANdb specified signals
  CANPack_SYSTEM_INFO_2 : canmsglib/CAN Pack  MsgList=(none)  MsgName=SYSTEM_INFO_2  MsgIDType=Extended (29-bit identifier)  MsgIdentifier=419387898  MsgLength=8  Remote=off  ApplyMinMax=off  BusOutput=on  SignalInfo={ 'system_info_2_1', '0', '8', 'LE', 'unsigned', 'Standard', '0', '1', '0', '0', '255'; 'system_info_2_2', '8', '8', 'LE', 'unsigned', 'Standard', '0', '1', '0', '0', '255'; 'system_info_2_3', '16', '8', 'LE', 'unsigned', 'Standard', '0', '1', '0', '0', '255'; 'system_info_2_4', '24', '8', 'LE', 'unsigned', 'Standard', '0', '1', '0', '0', '255'; 'system_info_2_5', '32', '8', 'LE', 'unsigned', 'Standard', '0', '1', '0', '0', '255'; 'system_info_2_6', '40', '8', 'LE', 'unsigned', 'Standard', '0', '1', '0', '0', '255'; 'system_info_2_7', '48', '8', 'LE', 'unsigned', 'Standard', '0', '1', '0', '0', '255'; 'system_info_2_8', '56', '8', 'LE', 'unsigned', 'Standard', '0', '1', '0', '0', '255' }
      settings: SourceProductBaseCode=ME,XP,VN  DataFormat=manually specified signals
  CANPack_SYSTEM_INFO_3 : canmsglib/CAN Pack  MsgList=(none)  MsgName=SYSTEM_INFO_3  MsgIDType=Extended (29-bit identifier)  MsgIdentifier=419389690  MsgLength=8  Remote=off  ApplyMinMax=off  BusOutput=on  SignalInfo={ 'system_info_3_1', '0', '8', 'LE', 'unsigned', 'Standard', '0', '1', '0', '0', '255'; 'system_info_3_2', '8', '8', 'LE', 'unsigned', 'Standard', '0', '1', '0', '0', '255'; 'system_info_3_3', '16', '8', 'LE', 'unsigned', 'Standard', '0', '1', '0', '0', '255'; 'system_info_3_4', '24', '8', 'LE', 'unsigned', 'Standard', '0', '1', '0', '0', '255'; 'system_info_3_5', '32', '8', 'LE', 'unsigned', 'Standard', '0', '1', '0', '0', '255'; 'system_info_3_6', '40', '8', 'LE', 'unsigned', 'Standard', '0', '1', '0', '0', '255'; 'system_info_3_7', '48', '8', 'LE', 'unsigned', 'Standard', '0', '1', '0', '0', '255'; 'system_info_3_8', '56', '8', 'LE', 'unsigned', 'Standard', '0', '1', '0', '0', '255' }
      settings: SourceProductBaseCode=ME,XP,VN  DataFormat=manually specified signals
  CANPack_SYSTEM_INFO_4 : canmsglib/CAN Pack  MsgList=(none)  MsgName=SYSTEM_INFO_4  MsgIDType=Extended (29-bit identifier)  MsgIdentifier=419389946  MsgLength=8  Remote=off  ApplyMinMax=off  BusOutput=on  SignalInfo={ 'system_info_4_1', '0', '16', 'LE', 'unsigned', 'Standard', '0', '1', '-32768', '0', '32767'; 'system_info_4_2', '16', '16', 'LE', 'unsigned', 'Standard', '0', '1', '0', '0', '65535'; 'system_info_4_3', '32', '16', 'LE', 'unsigned', 'Standard', '0', '1', '0', '0', '65535'; 'system_info_4_4', '48', '16', 'LE', 'unsigned', 'Standard', '0', '1', '0', '0', '65535' }
      settings: SourceProductBaseCode=ME,XP,VN  DataFormat=manually specified signals
  CANPack_SYSTEM_INFO_5 : canmsglib/CAN Pack  MsgList=(none)  MsgName=SYSTEM_INFO_5  MsgIDType=Extended (29-bit identifier)  MsgIdentifier=419390202  MsgLength=8  Remote=off  ApplyMinMax=off  BusOutput=on  SignalInfo={ 'system_info_5_1', '0', '16', 'LE', 'unsigned', 'Standard', '0', '1', '0', '0', '65535'; 'system_info_5_2', '16', '16', 'LE', 'unsigned', 'Standard', '0', '1', '0', '0', '65535'; 'system_info_5_3', '32', '16', 'LE', 'unsigned', 'Standard', '0', '1', '0', '0', '65535'; 'system_info_5_4', '48', '16', 'LE', 'unsigned', 'Standard', '0', '1', '0', '0', '65535' }
      settings: SourceProductBaseCode=ME,XP,VN  DataFormat=manually specified signals
  CANPack_hyd_Fluid_temp : canmsglib/CAN Pack  MsgList=(none)  MsgName=Log_AI_1  MsgIDType=Extended (29-bit identifier)  MsgIdentifier=402657831  MsgLength=8  Remote=off  ApplyMinMax=off  BusOutput=on  SignalInfo={ 'TrHydPumpDirectSens', '24', '8', 'LE', 'unsigned', 'Standard', '0', '1', '0', '0', '255'; 'TrHydPumpFilterClogSens', '8', '8', 'LE', 'unsigned', 'Standard', '0', '2', '0', '0', '510'; 'TrHydPumpSpeedSens1', '32', '8', 'LE', 'unsigned', 'Standard', '0', '50', '0', '0', '12750'; 'TrHydPumpSpeedSens2', '16', '8', 'LE', 'unsigned', 'Standard', '0', '50', '0', '0', '12750'; 'TrHydPumpTempSens', '40', '8', 'LE', 'unsigned', 'Standard', '0', '10', '0', '0', '2550'; 'TrHydPumpWasherTiltSens', '0', '8', 'LE', 'unsigned', 'Standard', '0', '20', '0', '0', '5100'; 'TransmissionMotorHydDistr', '48', '8', 'LE', 'unsigned', 'Standard', '0', '4', '0', '0', '1020' }
      settings: SourceProductBaseCode=ME,XP,VN  DataFormat=manually specified signals
  CANPack_hyd_Fluid_temp1 : canmsglib/CAN Pack  MsgList=(none)  MsgName=Log_AI_2  MsgIDType=Extended (29-bit identifier)  MsgIdentifier=402658087  MsgLength=8  Remote=off  ApplyMinMax=off  BusOutput=on  SignalInfo={ 'LowerGeneratorSignal', '56', '8', 'LE', 'unsigned', 'Standard', '0', '1', '0', '0', '255'; 'TrHydMotDirectSens', '16', '8', 'LE', 'unsigned', 'Standard', '0', '1', '0', '0', '255'; 'TrHydMotPressLineInForwardSens', '40', '8', 'LE', 'unsigned', 'Standard', '0', '100', '0', '0', '25500'; 'TrHydMotPressLineInReverseSens', '32', '8', 'LE', 'unsigned', 'Standard', '0', '100', '0', '0', '25500'; 'TrHydMotSpeedSens1', '0', '8', 'LE', 'unsigned', 'Standard', '0', '50', '0', '0', '12750'; 'TrHydMotSpeedSens2', '8', '8', 'LE', 'unsigned', 'Standard', '0', '50', '0', '0', '12750'; 'TrHydMotTempSens', '24', '8', 'LE', 'unsigned', 'Standard', '0', '10', '0', '0', '2550'; 'UpperGeneratorSignal', '48', '8', 'LE', 'unsigned', 'Standard', '0', '1', '0', '0', '255' }
      settings: SourceProductBaseCode=ME,XP,VN  DataFormat=manually specified signals
  CANPack_hyd_Fluid_temp2 : canmsglib/CAN Pack  MsgList=(none)  MsgName=Log_AI_3_Brake  MsgIDType=Extended (29-bit identifier)  MsgIdentifier=402658599  MsgLength=8  Remote=off  ApplyMinMax=off  BusOutput=on  SignalInfo={ 'BrkFrontCircPressSens', '16', '8', 'LE', 'unsigned', 'Standard', '0', '100', '0', '0', '25500'; 'BrkFrontSupplyCircPressSens', '40', '8', 'LE', 'unsigned', 'Standard', '0', '100', '0', '0', '25500'; 'BrkParkCircPressSens', '48', '8', 'LE', 'unsigned', 'Standard', '0', '100', '0', '0', '25500'; 'BrkParkSupplyCircPressSens', '24', '8', 'LE', 'unsigned', 'Standard', '0', '100', '0', '0', '25500'; 'BrkRearCircPressSens', '8', '8', 'LE', 'unsigned', 'Standard', '0', '100', '0', '0', '25500'; 'BrkRearSupplyCircPressSens', '32', '8', 'LE', 'unsigned', 'Standard', '0', '100', '0', '0', '25500'; 'StrAndBrkLSPressSens', '0', '8', 'LE', 'unsigned', 'Standard', '0', '100', '0', '0', '25500' }
      settings: SourceProductBaseCode=ME,XP,VN  DataFormat=manually specified signals
  CANPack_hyd_Fluid_temp3 : canmsglib/CAN Pack  MsgList=(none)  MsgName=Log_DI  MsgIDType=Extended (29-bit identifier)  MsgIdentifier=402658343  MsgLength=8  Remote=off  ApplyMinMax=off  BusOutput=on  SignalInfo={ 'ShutdownButtonSignal', '16', '2', 'LE', 'unsigned', 'Standard', '0', '1', '0', '0', '3'; 'TCHighGearIsActiveSens', '0', '2', 'LE', 'unsigned', 'Standard', '0', '1', '0', '0', '3'; 'TCLowGearIsActiveSens', '8', '2', 'LE', 'unsigned', 'Standard', '0', '1', '0', '0', '3' }
      settings: SourceProductBaseCode=ME,XP,VN  DataFormat=manually specified signals
  Constant31 : Constant  Commented=on  Value=pECANManual_BPNEnabler_Flag
  Constant32 : Constant  Commented=on  Value=pECANManual_BPNEnable
  Data Store Read : DataStoreRead  Commented=on  DataStoreName=DevicesControllerData  DataStoreElements=DevicesControllerData.ovc_permission
  Data Store Read1 : DataStoreRead  DataStoreName=LogInputInterfaceData  DataStoreElements=LogInputInterfaceData.AI_1_Log.log_transmPumpDirSens#LogInputInterfaceData.AI_1_Log.log_filterClogSens#LogInputInterfaceData.AI_1_Log.log_transPumpSpdSensSig1#LogInputInterfaceData.AI_1_Log.log_transPumpSpdSensSig2#LogInputInterfaceData.AI_1_Log.log_transPumpTempSens#LogInputInterfaceData.AI_1_Log.log_washerTiltPumpTransSens#LogInputInterfaceData.AI_1_Log.log_transPumpVlv
  Data Store Read10 : DataStoreRead  DataStoreName=LogInputInterfaceData  DataStoreElements=LogInputInterfaceData.SYSTEM_INFO_4.system_info_4_3
  Data Store Read11 : DataStoreRead  DataStoreName=LogInputInterfaceData  DataStoreElements=LogInputInterfaceData.SYSTEM_INFO_4.system_info_4_4
  Data Store Read12 : DataStoreRead  DataStoreName=LogInputInterfaceData  DataStoreElements=LogInputInterfaceData.SYSTEM_INFO_5.system_info_5_1
  Data Store Read13 : DataStoreRead  DataStoreName=LogInputInterfaceData  DataStoreElements=LogInputInterfaceData.SYSTEM_INFO_5.system_info_5_2
  Data Store Read14 : DataStoreRead  DataStoreName=LogInputInterfaceData  DataStoreElements=LogInputInterfaceData.SYSTEM_INFO_5.system_info_5_3
  Data Store Read15 : DataStoreRead  DataStoreName=LogInputInterfaceData  DataStoreElements=LogInputInterfaceData.SYSTEM_INFO_5.system_info_5_4
  Data Store Read16 : DataStoreRead  DataStoreName=LogInputInterfaceData  DataStoreElements=LogInputInterfaceData.SYSTEM_INFO_2.system_info_2_2
  Data Store Read17 : DataStoreRead  DataStoreName=LogInputInterfaceData  DataStoreElements=LogInputInterfaceData.SYSTEM_INFO_2.system_info_2_3
  Data Store Read18 : DataStoreRead  DataStoreName=LogInputInterfaceData  DataStoreElements=LogInputInterfaceData.SYSTEM_INFO_2.system_info_2_4
  Data Store Read19 : DataStoreRead  DataStoreName=LogInputInterfaceData  DataStoreElements=LogInputInterfaceData.SYSTEM_INFO_2.system_info_2_5
  Data Store Read2 : DataStoreRead  DataStoreName=LogInputInterfaceData  DataStoreElements=LogInputInterfaceData.AI_2_Log.log_transmMotDirSens#LogInputInterfaceData.AI_2_Log.log_hydMotPressLinePressSens#LogInputInterfaceData.AI_2_Log.log_reverseTransmMotPessLinePressSens#LogInputInterfaceData.AI_2_Log.log_transmHydMotSpdSensSig1#LogInputInterfaceData.AI_2_Log.log_transmHydMotSpdSensSig2#LogInputInterfaceData.AI_2_Log.log_hydMotTempSens
  Data Store Read20 : DataStoreRead  DataStoreName=LogInputInterfaceData  DataStoreElements=LogInputInterfaceData.SYSTEM_INFO_2.system_info_2_6
  Data Store Read21 : DataStoreRead  DataStoreName=LogInputInterfaceData  DataStoreElements=LogInputInterfaceData.SYSTEM_INFO_2.system_info_2_7
  Data Store Read22 : DataStoreRead  DataStoreName=LogInputInterfaceData  DataStoreElements=LogInputInterfaceData.SYSTEM_INFO_2.system_info_2_8
  Data Store Read23 : DataStoreRead  DataStoreName=LogInputInterfaceData  DataStoreElements=LogInputInterfaceData.SYSTEM_INFO_3.system_info_3_1
  Data Store Read24 : DataStoreRead  DataStoreName=LogInputInterfaceData  DataStoreElements=LogInputInterfaceData.SYSTEM_INFO_3.system_info_3_2
  Data Store Read25 : DataStoreRead  DataStoreName=LogInputInterfaceData  DataStoreElements=LogInputInterfaceData.SYSTEM_INFO_3.system_info_3_3
  Data Store Read26 : DataStoreRead  DataStoreName=LogInputInterfaceData  DataStoreElements=LogInputInterfaceData.SYSTEM_INFO_3.system_info_3_4
  Data Store Read27 : DataStoreRead  DataStoreName=LogInputInterfaceData  DataStoreElements=LogInputInterfaceData.SYSTEM_INFO_3.system_info_3_5
  Data Store Read28 : DataStoreRead  DataStoreName=LogInputInterfaceData  DataStoreElements=LogInputInterfaceData.SYSTEM_INFO_3.system_info_3_6
  Data Store Read29 : DataStoreRead  DataStoreName=LogInputInterfaceData  DataStoreElements=LogInputInterfaceData.SYSTEM_INFO_3.system_info_3_7
  Data Store Read3 : DataStoreRead  DataStoreName=LogInputInterfaceData  DataStoreElements=LogInputInterfaceData.AI_3_Log.log_brkFrontCircPressSens#LogInputInterfaceData.AI_3_Log.log_brkSupplyFrontPressSens#LogInputInterfaceData.AI_3_Log.drainParkPressSens#LogInputInterfaceData.AI_3_Log.log_brkSupplyParkPressSens#LogInputInterfaceData.AI_3_Log.log_brkRearCircPressSens#LogInputInterfaceData.AI_3_Log.log_brkSupplyRearPressSens#LogInputInterfaceData.AI_3_Log.log_steeringLSPressSens
  Data Store Read30 : DataStoreRead  DataStoreName=LogInputInterfaceData  DataStoreElements=LogInputInterfaceData.SYSTEM_INFO_3.system_info_3_8
  Data Store Read4 : DataStoreRead  DataStoreName=LogInputInterfaceData  DataStoreElements=LogInputInterfaceData.DI_Log.log_lowerGenWorkSig
  Data Store Read5 : DataStoreRead  DataStoreName=LogInputInterfaceData  DataStoreElements=LogInputInterfaceData.DI_Log.log_upperGenWorkSig
  Data Store Read6 : DataStoreRead  DataStoreName=LogInputInterfaceData  DataStoreElements=LogInputInterfaceData.DI_Log.log_shutdownButtonSig#LogInputInterfaceData.DI_Log.log_transCaseHighGearIsActiveSens#LogInputInterfaceData.DI_Log.log_transCaseLowGearIsActiveSens
  Data Store Read7 : DataStoreRead  DataStoreName=LogInputInterfaceData  DataStoreElements=LogInputInterfaceData.SYSTEM_INFO_4.system_info_4_1
  Data Store Read8 : DataStoreRead  DataStoreName=LogInputInterfaceData  DataStoreElements=LogInputInterfaceData.SYSTEM_INFO_2.system_info_2_1
  Data Store Read9 : DataStoreRead  DataStoreName=LogInputInterfaceData  DataStoreElements=LogInputInterfaceData.SYSTEM_INFO_4.system_info_4_2
  Data Type Conversion{3,6..20} (16 alike) : DataTypeConversion  OutDataTypeStr=uint8
  Data Type Conversion21 : DataTypeConversion  OutDataTypeStr=int16
  Data Type Conversion{22..28} (7 alike) : DataTypeConversion  OutDataTypeStr=uint16
  Function Caller2 : FunctionCaller  FunctionPrototype=rawValue = convDIOSttTypeToNum(enumValue)  InputArgumentSpecifications=<Enter example>  OutputArgumentSpecifications=<Enter example>
  Function Caller3 : FunctionCaller  FunctionPrototype=rawValue = convDIOSttTypeToNum(enumValue)  InputArgumentSpecifications=<Enter example>  OutputArgumentSpecifications=<Enter example>
  Function Caller4 : FunctionCaller  FunctionPrototype=rawValue = convDIOSttTypeToNum(enumValue)  InputArgumentSpecifications=<Enter example>  OutputArgumentSpecifications=<Enter example>
  MATLAB Function6 : MATLAB Function  Commented=on  TreatAsAtomicUnit=on
  Multiport Switch5 : MultiPortSwitch  Commented=on  DataPortOrder=Zero-based contiguous  Inputs=2  zeroidx=on
  Terminator : Terminator  Commented=on
  Terminator{1..8} (8 alike) : Terminator
  transmit_message_dcdc_in_control : TTlibrary/CAN/transmit_message_name  Commented=on  channel=IO_CAN_CHANNEL_0  id_format=IO_CAN_STD_FRAME  retranslation=off  io_error=on  sample_time=-1
      settings: SourceProductName=TT control 500 series
  transmit_message_hyd_fluid_temp{,1..3} (4 alike) : TTlibrary/CAN/transmit_message_name  channel=IO_CAN_CHANNEL_6  id_format=IO_CAN_EXT_FRAME  retranslation=off  io_error=on  sample_time=-1
      settings: SourceProductName=TT control 500 series
  transmit_system_info_{2..5} (4 alike) : TTlibrary/CAN/transmit_message_name  channel=IO_CAN_CHANNEL_6  id_format=IO_CAN_EXT_FRAME  retranslation=off  io_error=on  sample_time=-1
      settings: SourceProductName=TT control 500 series
  wires:
  Data Type Conversion27/1 -> CANPack_SYSTEM_INFO_5/3
  CANPack_SYSTEM_INFO_5/1 -> transmit_system_info_5/1
  Constant32/1 -> Multiport Switch5/3
  CANPack_DCDC_IN_Control/1 -> transmit_message_dcdc_in_control/1
  Data Type Conversion16/1 -> CANPack_SYSTEM_INFO_3/1
  transmit_system_info_3/1 -> Terminator2/1  "error_tx_transmit_system_info_3"
  Abs10/1 -> Data Type Conversion26/1
  Data Type Conversion10/1 -> CANPack_SYSTEM_INFO_2/6
  Data Type Conversion20/1 -> CANPack_SYSTEM_INFO_3/5
  Data Store Read2/6 -> CANPack_hyd_Fluid_temp1/7
  Data Type Conversion25/1 -> CANPack_SYSTEM_INFO_5/1
  CANPack_hyd_Fluid_temp1/1 -> transmit_message_hyd_fluid_temp1/1
  transmit_system_info_2/1 -> Terminator1/1  "error_tx_transmit_system_info_2"
  CANPack_SYSTEM_INFO_3/1 -> transmit_system_info_3/1
  Data Type Conversion8/1 -> CANPack_SYSTEM_INFO_2/4
  Data Type Conversion21/1 -> CANPack_SYSTEM_INFO_4/1
  Data Type Conversion7/1 -> CANPack_SYSTEM_INFO_2/3
  transmit_message_dcdc_in_control/1 -> Terminator/1  "error_tx_transmit_message_dcdc_in_control"
  Data Type Conversion9/1 -> CANPack_SYSTEM_INFO_2/5
  Data Type Conversion19/1 -> CANPack_SYSTEM_INFO_3/4
  Data Store Read6/2 -> Function Caller3/1
  Data Type Conversion17/1 -> CANPack_SYSTEM_INFO_3/2
  CANPack_hyd_Fluid_temp3/1 -> transmit_message_hyd_fluid_temp3/1
  Data Store Read1/3 -> CANPack_hyd_Fluid_temp/3
  transmit_message_hyd_fluid_temp1/1 -> Terminator4/1  "error_tx_transmit_message_hyd_fluid_temp1"
  transmit_message_hyd_fluid_temp/1 -> Terminator3/1  "error_tx_transmit_message_hyd_fluid_temp"
  Function Caller2/1 -> CANPack_hyd_Fluid_temp3/1
  Constant31/1 -> Multiport Switch5/1
  Data Type Conversion28/1 -> CANPack_SYSTEM_INFO_5/4
  Data Type Conversion3/1 -> CANPack_SYSTEM_INFO_2/1
  CANPack_SYSTEM_INFO_4/1 -> transmit_system_info_4/1
  Data Type Conversion15/1 -> CANPack_SYSTEM_INFO_3/8
  Data Store Read1/6 -> CANPack_hyd_Fluid_temp/6
  CANPack_hyd_Fluid_temp/1 -> transmit_message_hyd_fluid_temp/1
  Data Store Read5/1 -> CANPack_hyd_Fluid_temp1/8
  Data Type Conversion18/1 -> CANPack_SYSTEM_INFO_3/3
  Data Store Read9/1 -> Data Type Conversion22/1
  Data Type Conversion11/1 -> CANPack_SYSTEM_INFO_2/7
  CANPack_hyd_Fluid_temp2/1 -> transmit_message_hyd_fluid_temp2/1
  Data Store Read2/1 -> CANPack_hyd_Fluid_temp1/2
  Data Type Conversion23/1 -> CANPack_SYSTEM_INFO_4/3
  Data Store Read3/4 -> CANPack_hyd_Fluid_temp2/4
  Data Store Read3/7 -> CANPack_hyd_Fluid_temp2/7
  Data Store Read1/5 -> CANPack_hyd_Fluid_temp/5
  Data Store Read2/4 -> CANPack_hyd_Fluid_temp1/5
  transmit_message_hyd_fluid_temp2/1 -> Terminator5/1  "error_tx_transmit_message_hyd_fluid_temp2"
  Function Caller3/1 -> CANPack_hyd_Fluid_temp3/2
  Function Caller4/1 -> CANPack_hyd_Fluid_temp3/3
  Abs12/1 -> Data Type Conversion28/1
  Data Type Conversion22/1 -> CANPack_SYSTEM_INFO_4/2
  Data Type Conversion12/1 -> CANPack_SYSTEM_INFO_2/8
  Data Store Read3/6 -> CANPack_hyd_Fluid_temp2/6
  Data Store Read1/4 -> CANPack_hyd_Fluid_temp/4
  Data Store Read7/1 -> Data Type Conversion21/1
  Abs11/1 -> Data Type Conversion27/1
  CANPack_SYSTEM_INFO_2/1 -> transmit_system_info_2/1
  Data Store Read27/1 -> Data Type Conversion20/1
  Data Type Conversion24/1 -> CANPack_SYSTEM_INFO_4/4
  Data Store Read19/1 -> Data Type Conversion9/1
  Data Store Read20/1 -> Data Type Conversion10/1
  Data Type Conversion14/1 -> CANPack_SYSTEM_INFO_3/7
  Data Store Read13/1 -> Abs10/1
  transmit_system_info_5/1 -> Terminator7/1  "error_tx_transmit_system_info_5"
  Data Type Conversion13/1 -> CANPack_SYSTEM_INFO_3/6
  Data Store Read3/1 -> CANPack_hyd_Fluid_temp2/1
  Data Store Read4/1 -> CANPack_hyd_Fluid_temp1/1
  Data Store Read8/1 -> Data Type Conversion3/1
  Data Store Read15/1 -> Abs12/1
  Data Store Read3/5 -> CANPack_hyd_Fluid_temp2/5
  Data Store Read14/1 -> Abs11/1
  Data Store Read1/1 -> CANPack_hyd_Fluid_temp/1
  Data Store Read3/3 -> CANPack_hyd_Fluid_temp2/3
  Data Store Read1/7 -> CANPack_hyd_Fluid_temp/7
  Abs8/1 -> Data Type Conversion24/1
  Data Store Read12/1 -> Abs9/1
  Data Store Read16/1 -> Data Type Conversion6/1
  Data Store Read23/1 -> Data Type Conversion16/1
  Abs9/1 -> Data Type Conversion25/1
  Data Store Read2/3 -> CANPack_hyd_Fluid_temp1/4
  Data Store Read26/1 -> Data Type Conversion19/1
  Multiport Switch5/1 -> CANPack_DCDC_IN_Control/1
  Data Store Read22/1 -> Data Type Conversion12/1
  Data Store Read25/1 -> Data Type Conversion18/1
  Data Store Read21/1 -> Data Type Conversion11/1
  Data Store Read2/2 -> CANPack_hyd_Fluid_temp1/3
  Data Store Read17/1 -> Data Type Conversion7/1
  Data Store Read6/1 -> Function Caller2/1
  Data Store Read28/1 -> Data Type Conversion13/1
  Data Store Read1/2 -> CANPack_hyd_Fluid_temp/2
  Data Store Read6/3 -> Function Caller4/1
  Data Store Read29/1 -> Data Type Conversion14/1
  Data Store Read10/1 -> Data Type Conversion23/1
  MATLAB Function6/1(value) -> Multiport Switch5/2
  Data Store Read11/1 -> Abs8/1
  Data Store Read18/1 -> Data Type Conversion8/1
  transmit_system_info_4/1 -> Terminator6/1  "error_tx_transmit_system_info_4"
  transmit_message_hyd_fluid_temp3/1 -> Terminator8/1  "error_tx_transmit_message_hyd_fluid_temp3"
  Data Store Read/1 -> MATLAB Function6/1(input)
  Data Store Read3/2 -> CANPack_hyd_Fluid_temp2/2
  Data Store Read24/1 -> Data Type Conversion17/1
  Data Store Read30/1 -> Data Type Conversion15/1
  Data Store Read2/5 -> CANPack_hyd_Fluid_temp1/6
  Data Type Conversion26/1 -> CANPack_SYSTEM_INFO_5/2
  Data Type Conversion6/1 -> CANPack_SYSTEM_INFO_2/2
